simulink model "LaneChangeRoad2B_Disp"  (R2017b)
settings: Solver=FixedStepDiscrete  StartTime=0.0  StopTime=80  FixedStep=0.001  RelTol=1e-3
PostLoadFcn:
  | load vehStateObject.mat;
undefined symbols (not defined in the file or in its folder): magnitude
libraries: simulink x8, Solver_SF x1
settings Model: Creator=Lenovo  LastModifiedBy=Lenovo

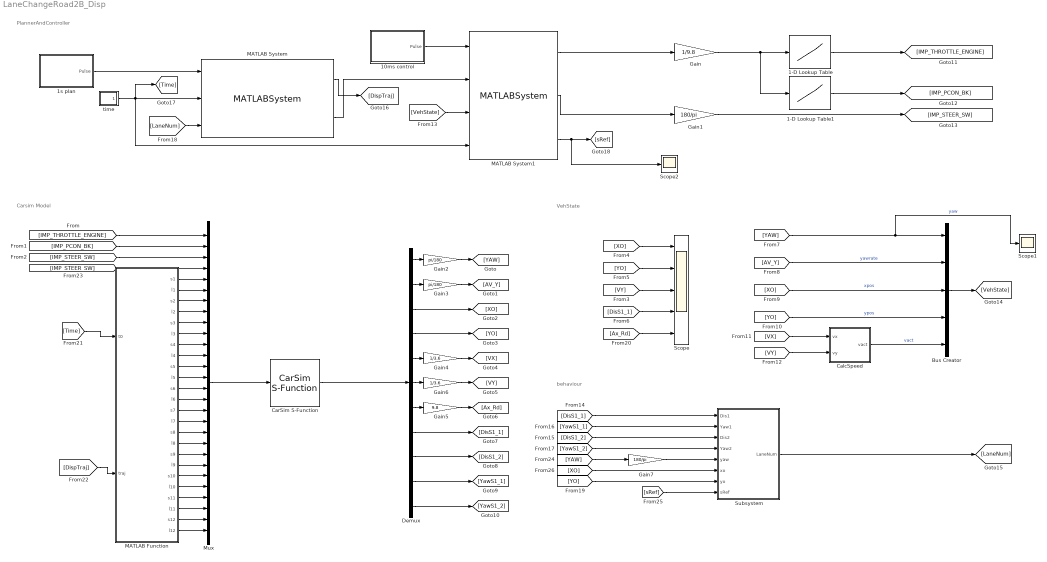
== system LaneChangeRoad2B_Disp ==
  note: behaviour
  note: VehState
  note: Carsim Model
  note: PlannerAndController
  1-D Lookup Table : Lookup_n-D  NumberOfTableDimensions=1  BreakpointsForDimension1=[-0.028, -0.023, -0.017, -0.012, -0.0075, -0.0035, 0.0005, 0.0085, 0.016,0.04, 0.125, 0.45]  Table=[0, 0.01, 0.02, 0.03, 0.04, 0.05, 0.06, 0.08, 0.1, 0.11, 0.15, 1]  ExtrapMethod=Clip  InternalRulePriority=Speed  RndMeth=Simplest  InputSameDT=on
  1-D Lookup Table1 : Lookup_n-D  NumberOfTableDimensions=1  BreakpointsForDimension1=[-0.175,-0.13,-0.0875,-0.073,-0.057,-0.045,-0.028]  Table=[1,0.7, 0.4, 0.3, 0.2, 0.1, 0]  ExtrapMethod=Clip  InternalRulePriority=Speed  RndMeth=Simplest  InputSameDT=on
  10ms control : Subsystem
  1s plan : Subsystem
  Bus Creator : BusCreator  Inputs=5  OutDataTypeStr=Bus: VehStateObject
  CalcSpeed : Subsystem
  CarSim S-Function : Solver_SF/CarSim S-Function  Priority=1  SIMFILE=simfile.sim  Run_RTs=off  vs_state_ind=Run  StopMode_ind=Vehicle Model
  Demux : Demux  Outputs=11
  Gain : Gain  Gain=1/9.8
  Gain1 : Gain  Gain=180/pi
  Gain2 : Gain  Gain=pi/180
  Gain3 : Gain  Gain=pi/180
  Gain4 : Gain  Gain=1/3.6
  Gain5 : Gain  Gain=9.8
  Gain6 : Gain  Gain=1/3.6
  Gain7 : Gain  Gain=180/pi
  MATLAB Function : MATLAB Function  TreatAsAtomicUnit=on
  MATLAB System : MATLABSystem  System=LaneChangePlanner2  SimulateUsing=Interpreted execution
      mask Type: LaneChangePlanner2
      mask Display:
      | disp('LaneChangePlanner2');
      | port_label('input',1,'replanflag');
      | port_label('input',2,'t0');
      | port_label('input',3,'lanenum');
      | port_label('output',1,'trajDisp');
      | port_label('output',2,'trajRet');
  MATLAB System1 : MATLABSystem  System=MPCControlB  SimulateUsing=Interpreted execution
      mask Type: MPCControlB
      mask Display:
      | disp('MPCControlB');
      | port_label('input',1,'controlFlag');
      | port_label('input',2,'traj_ref');
      | port_label('input',3,'veh_state');
      | port_label('input',4,'t');
      | port_label('output',1,'acc');
      | port_label('output',2,'steer');
      | port_label('output',3,'sRef');
  Mux : Mux  Inputs=28
  Scope : Scope  NumInputPorts=5
  Scope1 : Scope
  Scope2 : Scope
  Subsystem : Subsystem
  time : Subsystem
  wires:
  CarSim S-Function/1 -> Demux/1
  Mux/1 -> CarSim S-Function/1
  Demux/1 -> Gain2/1
  Demux/2 -> Gain3/1
  Demux/3 -> [XO]
  Demux/4 -> [YO]
  Demux/5 -> Gain4/1
  Demux/6 -> Gain6/1
  Demux/7 -> Gain5/1
  Demux/8 -> [DisS1_1]
  Demux/9 -> [DisS1_2]
  1-D Lookup Table/1 -> [IMP_THROTTLE_ENGINE]
  1-D Lookup Table1/1 -> [IMP_PCON_BK]
  [XO] -> Scope/1
  [YO] -> Scope/2
  [VY] -> Scope/3
  [DisS1_1] -> Scope/4
  1s plan/1(Pulse) -> MATLAB System/1
  MATLAB System/1 -> [DispTraj]
  [LaneNum] -> MATLAB System/3
  MATLAB System1/1 -> Gain/1
  MATLAB System1/2 -> Gain1/1
  Gain/1 -> 1-D Lookup Table1/1, 1-D Lookup Table/1
  Gain1/1 -> [IMP_STEER_SW]
  [YO] -> Bus Creator/4  "ypos"
  [XO] -> Bus Creator/3  "xpos"
  [AV_Y] -> Bus Creator/2  "yawrate"
  [YAW] -> Scope1/1, Bus Creator/1  "yaw"
  Bus Creator/1 -> [VehState]
  [VehState] -> MATLAB System1/3
  time/1(Time) -> [Time], MATLAB System1/4, MATLAB System/2
  10ms control/1(Pulse) -> MATLAB System1/1
  [DisS1_1] -> Subsystem/1(Dis1)
  [YawS1_1] -> Subsystem/2(Yaw1)
  [DisS1_2] -> Subsystem/3(Dis2)
  [YawS1_2] -> Subsystem/4(Yaw2)
  Subsystem/1(LaneNum) -> [LaneNum]
  [VX] -> CalcSpeed/1(vx)
  [VY] -> CalcSpeed/2(vy)
  CalcSpeed/1(vact) -> Bus Creator/5  "vact"
  [YO] -> Subsystem/7(yo)
  Gain2/1 -> [YAW]
  Gain3/1 -> [AV_Y]
  Gain4/1 -> [VX]
  Gain5/1 -> [Ax_Rd]
  Gain6/1 -> [VY]
  Demux/10 -> [YawS1_1]
  Demux/11 -> [YawS1_2]
  [Ax_Rd] -> Scope/5
  [Time] -> MATLAB Function/1(t0)
  [DispTraj] -> MATLAB Function/2(traj)
  MATLAB System/2 -> MATLAB System1/2
  [IMP_THROTTLE_ENGINE] -> Mux/1
  [IMP_PCON_BK] -> Mux/2
  [IMP_STEER_SW] -> Mux/3
  [IMP_STEER_SW] -> Mux/4
  MATLAB Function/1(s1) -> Mux/5
  MATLAB Function/2(l1) -> Mux/6
  MATLAB Function/3(s2) -> Mux/7
  MATLAB Function/4(l2) -> Mux/8
  MATLAB Function/5(s3) -> Mux/9
  MATLAB Function/6(l3) -> Mux/10
  MATLAB Function/7(s4) -> Mux/11
  MATLAB Function/8(l4) -> Mux/12
  MATLAB Function/9(s5) -> Mux/13
  MATLAB Function/10(l5) -> Mux/14
  MATLAB Function/11(s6) -> Mux/15
  MATLAB Function/12(l6) -> Mux/16
  MATLAB Function/13(s7) -> Mux/17
  MATLAB Function/14(l7) -> Mux/18
  MATLAB Function/15(s8) -> Mux/19
  MATLAB Function/16(l8) -> Mux/20
  MATLAB Function/17(s9) -> Mux/21
  MATLAB Function/18(l9) -> Mux/22
  MATLAB Function/19(s10) -> Mux/23
  MATLAB Function/20(l10) -> Mux/24
  MATLAB Function/21(s11) -> Mux/25
  MATLAB Function/22(l11) -> Mux/26
  MATLAB Function/23(s12) -> Mux/27
  MATLAB Function/24(l12) -> Mux/28
  [YAW] -> Gain7/1
  Gain7/1 -> Subsystem/5(yaw)
  MATLAB System1/3 -> Scope2/1, [sRef]
  [sRef] -> Subsystem/8(sRef)
  [XO] -> Subsystem/6(xo)

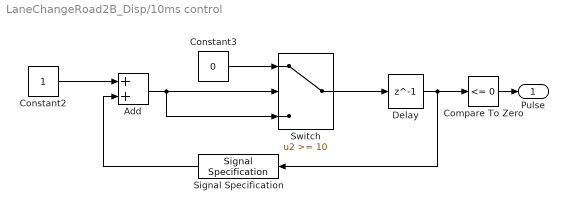
== system LaneChangeRoad2B_Disp/10ms control ==
  Add : Sum
  Compare To Zero : simulink/Logic and Bit Operations/Compare To Zero  relop=<=  OutDataTypeStr=boolean
  Constant2 : Constant
  Constant3 : Constant  Value=0
  Delay : Delay  DelayLength=1
  Signal Specification : SignalSpecification  SampleTime=0.001
  Switch : Switch  Threshold=10
  Pulse : Outport
  wires:
  Constant3/1 -> Switch/1
  Constant2/1 -> Add/1
  Switch/1 -> Delay/1
  Compare To Zero/1 -> Pulse/1
  Add/1 -> Switch/2, Switch/3
  Delay/1 -> Signal Specification/1, Compare To Zero/1
  Signal Specification/1 -> Add/2

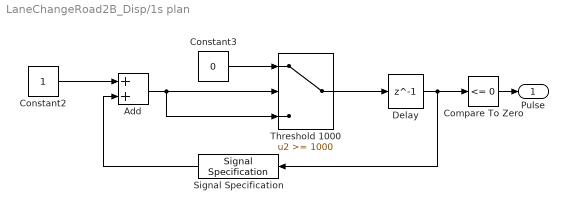
== system LaneChangeRoad2B_Disp/1s plan ==
  Add : Sum
  Compare To Zero : simulink/Logic and Bit Operations/Compare To Zero  relop=<=  OutDataTypeStr=boolean
  Constant2 : Constant
  Constant3 : Constant  Value=0
  Delay : Delay  DelayLength=1
  Signal Specification : SignalSpecification  SampleTime=0.001
  Threshold 1000 : Switch  Threshold=1000
  Pulse : Outport
  wires:
  Signal Specification/1 -> Add/2
  Delay/1 -> Compare To Zero/1, Signal Specification/1
  Add/1 -> Threshold 1000/3, Threshold 1000/2
  Compare To Zero/1 -> Pulse/1
  Threshold 1000/1 -> Delay/1
  Constant2/1 -> Add/1
  Constant3/1 -> Threshold 1000/1

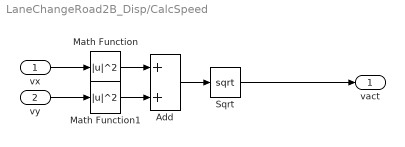
== system LaneChangeRoad2B_Disp/CalcSpeed ==
  vx : Inport
  vy : Inport  Port=2
  Add : Sum
  Math Function : Math  Operator=magnitude^2  SaturateOnIntegerOverflow=on
  Math Function1 : Math  Operator=magnitude^2  SaturateOnIntegerOverflow=on
  Sqrt : Sqrt  SaturateOnIntegerOverflow=on
  vact : Outport
  wires:
  Math Function1/1 -> Add/2
  Sqrt/1 -> vact/1
  vx/1 -> Math Function/1
  vy/1 -> Math Function1/1
  Add/1 -> Sqrt/1
  Math Function/1 -> Add/1

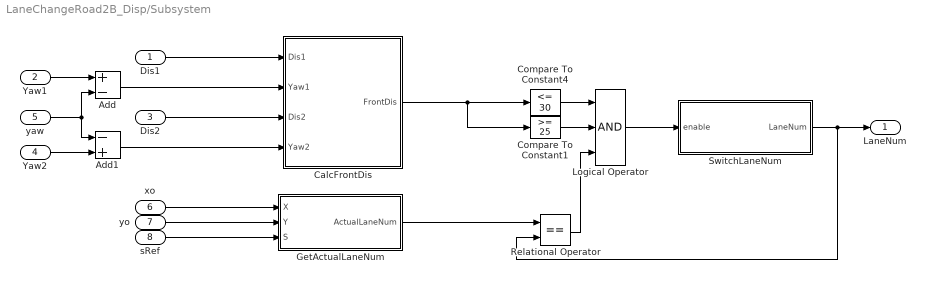
== system LaneChangeRoad2B_Disp/Subsystem ==
  Dis1 : Inport
  Yaw1 : Inport  Port=2
  Dis2 : Inport  Port=3
  Yaw2 : Inport  Port=4
  yaw : Inport  Port=5
  xo : Inport  Port=6
  yo : Inport  Port=7
  sRef : Inport  Port=8  OutDataTypeStr=double  PortDimensions=[1,1]
  Add : Sum  Inputs=+-
  Add1 : Sum  Inputs=-+
  CalcFrontDis : Subsystem
  Compare To Constant1 : simulink/Logic and Bit Operations/Compare To Constant  relop=>=  const=25  OutDataTypeStr=boolean
  Compare To Constant4 : simulink/Logic and Bit Operations/Compare To Constant  relop=<=  const=30  OutDataTypeStr=boolean
  GetActualLaneNum : Subsystem
  Logical Operator : Logic  Inputs=3  AllPortsSameDT=off  OutDataTypeStr=boolean
  Relational Operator : RelationalOperator  Operator===  OutDataTypeStr=boolean  RndMeth=Simplest
  SwitchLaneNum : Subsystem
  LaneNum : Outport
  wires:
  Dis1/1 -> CalcFrontDis/1(Dis1)
  Add/1 -> CalcFrontDis/2(Yaw1)
  Dis2/1 -> CalcFrontDis/3(Dis2)
  Add1/1 -> CalcFrontDis/4(Yaw2)
  CalcFrontDis/1(FrontDis) -> Compare To Constant1/1, Compare To Constant4/1
  GetActualLaneNum/1(ActualLaneNum) -> Relational Operator/1
  Compare To Constant4/1 -> Logical Operator/1
  Relational Operator/1 -> Logical Operator/3
  Logical Operator/1 -> SwitchLaneNum/1(enable)
  SwitchLaneNum/1(LaneNum) -> LaneNum/1, Relational Operator/2
  Yaw1/1 -> Add/1
  yaw/1 -> Add1/1, Add/2
  Yaw2/1 -> Add1/2
  xo/1 -> GetActualLaneNum/1(X)
  yo/1 -> GetActualLaneNum/2(Y)
  sRef/1 -> GetActualLaneNum/3(S)
  Compare To Constant1/1 -> Logical Operator/2

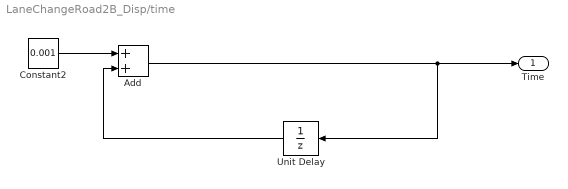
== system LaneChangeRoad2B_Disp/time ==
  Add : Sum
  Constant2 : Constant  Value=0.001
  Unit Delay : UnitDelay  SampleTime=-1
  Time : Outport
  wires:
  Constant2/1 -> Add/1
  Add/1 -> Time/1, Unit Delay/1
  Unit Delay/1 -> Add/2

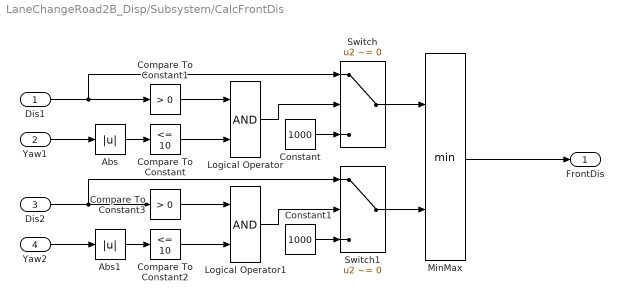
== system LaneChangeRoad2B_Disp/Subsystem/CalcFrontDis ==
  Dis1 : Inport
  Yaw1 : Inport  Port=2
  Dis2 : Inport  Port=3
  Yaw2 : Inport  Port=4
  Abs : Abs
  Abs1 : Abs
  Compare To Constant : simulink/Logic and Bit Operations/Compare To Constant  relop=<=  const=10  OutDataTypeStr=boolean
  Compare To Constant1 : simulink/Logic and Bit Operations/Compare To Constant  relop=>  const=0  OutDataTypeStr=boolean
  Compare To Constant2 : simulink/Logic and Bit Operations/Compare To Constant  relop=<=  const=10  OutDataTypeStr=boolean
  Compare To Constant3 : simulink/Logic and Bit Operations/Compare To Constant  relop=>  const=0  OutDataTypeStr=boolean
  Constant : Constant  Value=1000
  Constant1 : Constant  Value=1000
  Logical Operator : Logic  AllPortsSameDT=off  OutDataTypeStr=boolean
  Logical Operator1 : Logic  AllPortsSameDT=off  OutDataTypeStr=boolean
  MinMax : MinMax  Inputs=2
  Switch : Switch  Criteria=u2 ~= 0
  Switch1 : Switch  Criteria=u2 ~= 0
  FrontDis : Outport
  wires:
  Yaw2/1 -> Abs1/1
  Abs/1 -> Compare To Constant/1
  Dis2/1 -> Compare To Constant3/1, Switch1/1
  Compare To Constant1/1 -> Logical Operator/1
  Abs1/1 -> Compare To Constant2/1
  Compare To Constant2/1 -> Logical Operator1/2
  Switch/1 -> MinMax/1
  Constant/1 -> Switch/3
  Compare To Constant3/1 -> Logical Operator1/1
  Dis1/1 -> Switch/1, Compare To Constant1/1
  MinMax/1 -> FrontDis/1
  Switch1/1 -> MinMax/2
  Compare To Constant/1 -> Logical Operator/2
  Logical Operator1/1 -> Switch1/2
  Logical Operator/1 -> Switch/2
  Constant1/1 -> Switch1/3
  Yaw1/1 -> Abs/1

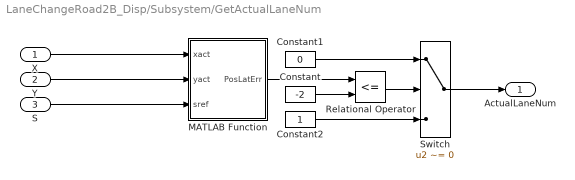
== system LaneChangeRoad2B_Disp/Subsystem/GetActualLaneNum ==
  X : Inport
  Y : Inport  Port=2
  S : Inport  Port=3
  Constant : Constant  Value=-2
  Constant1 : Constant  Value=0
  Constant2 : Constant
  MATLAB Function : MATLAB Function  TreatAsAtomicUnit=on
  Relational Operator : RelationalOperator  Operator=<=  OutDataTypeStr=boolean  RndMeth=Simplest
  Switch : Switch  Criteria=u2 ~= 0
  ActualLaneNum : Outport
  wires:
  X/1 -> MATLAB Function/1(xact)
  Y/1 -> MATLAB Function/2(yact)
  S/1 -> MATLAB Function/3(sref)
  MATLAB Function/1(PosLatErr) -> Relational Operator/1
  Relational Operator/1 -> Switch/2
  Switch/1 -> ActualLaneNum/1
  Constant/1 -> Relational Operator/2
  Constant1/1 -> Switch/1
  Constant2/1 -> Switch/3

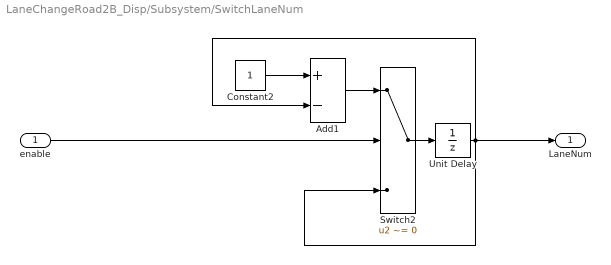
== system LaneChangeRoad2B_Disp/Subsystem/SwitchLaneNum ==
  enable : Inport
  Add1 : Sum  Inputs=+-
  Constant2 : Constant
  Switch2 : Switch  Criteria=u2 ~= 0
  Unit Delay : UnitDelay  InitialCondition=1  SampleTime=-1
  LaneNum : Outport
  wires:
  Switch2/1 -> Unit Delay/1
  Add1/1 -> Switch2/1
  Unit Delay/1 -> LaneNum/1, Add1/2, Switch2/3
  enable/1 -> Switch2/2
  Constant2/1 -> Add1/1

== matlab function LaneChangeRoad2B_Disp/Subsystem/GetActualLaneNum/MATLAB Function ==
  data: xact input size=[1,1]; yact input size=[1,1]; sref input size=[1,1]; PosLatErr output size=[1,1]
function PosLatErr = fcn(xact, yact, sref)
mat = load('roadpointdata.mat');
xs = mat.pointdata(:,1);
ys = mat.pointdata(:,2);
phis = mat.pointdata(:,3);
ss = mat.pointdata(:,6);
xref = interp1(ss, xs , sref);
yref = interp1(ss, ys , sref);
phiref = interp1(ss, phis , sref);
PosLatErr = (yref-yact)*cos(phiref)-(xref-xact)*sin(phiref);

== matlab function LaneChangeRoad2B_Disp/MATLAB Function ==
  data: t0 input; s1 output; traj input; l1 output; s2 output; l2 output; s3 output; l3 output; s4 output; l4 output; s5 output; l5 output; s6 output; l6 output; s7 output; l7 output; s8 output; l8 output; s9 output; l9 output; s10 output; l10 output; s11 output; l11 output; s12 output; l12 output
function [s1,l1,s2,l2,s3,l3,s4,l4,s5,l5,s6,l6,s7,l7,s8,l8,s9,l9,s10,l10,s11,l11,s12,l12] = GetDispTrajPoint(t0, traj)
selectIdx = 1;
for i = 1:size(traj,1)
    if abs(t0 - traj(i,3)) <= 0.0001
        selectIdx = i;
        break;
    end
end
step = 40;
idx = step;
s1 = traj(selectIdx + idx ,1);
l1 = traj(selectIdx + idx,2);

idx = idx + step;
s2 = traj(selectIdx + idx,1);
l2 = traj(selectIdx + idx,2);

idx = idx + step;
s3 = traj(selectIdx + idx,1);
l3 = traj(selectIdx + idx,2);

idx = idx + step;
s4 = traj(selectIdx + idx,1);
l4 = traj(selectIdx + idx,2);

idx = idx + step;
s5 = traj(selectIdx + idx,1);
l5 = traj(selectIdx + idx,2);

idx = idx + step;
s6 = traj(selectIdx + idx,1);
l6 = traj(selectIdx + idx,2);

idx = idx + step;
s7 = traj(selectIdx + idx,1);
l7 = traj(selectIdx + idx,2);

idx = idx + step;
s8 = traj(selectIdx + idx,1);
l8 = traj(selectIdx + idx,2);

idx = idx + step;
s9 = traj(selectIdx + idx,1);
l9 = traj(selectIdx + idx,2);

idx = idx + step;
s10 = traj(selectIdx + idx,1);
l10= traj(selectIdx + idx,2);

idx = idx + step;
s11 = traj(selectIdx + idx,1);
l11= traj(selectIdx + idx,2);

idx = idx + step;
s12 = traj(selectIdx + idx,1);
l12= traj(selectIdx + idx,2);
